simulink model "openloop_response"  (R2022b)
settings: Solver=ode15s  StartTime=0.0  StopTime=20  RelTol=1e-7  AbsTol=1e-7  EnableMultiTasking=on
InitFcn:
  | datacstr
values from neighbouring files (symbols this model uses):
  c_bar = 0.5    [main.m]
  T_bar = 350    [main.m]
libraries: simulink x1
settings Model: Creator=scattolini  LastModifiedBy=marco
settings SolverCC: AutoScaleAbsTol=off  AlgebraicLoopSolver=TrustRegion
settings DataIOCC: SaveFormat=Array  SignalLoggingSaveFormat=ModelDataLogs  ReturnWorkspaceOutputs=off  SignalLoggingName=sigsOut
settings OptimizationCC: BlockReduction=off  BooleanDataType=off  DefaultParameterBehavior=Inlined  BufferReuse=off  ExpressionDepthLimit=2147483647  InitFltsAndDblsToZero=on  LifeSpan=inf
settings DebuggingCC: SaveWithParameterizedLinksMsg=none  UnderspecifiedInitializationDetection=Classic  MergeDetectMultiDrivingBlocksExec=none  SignalResolutionControl=TryResolveAllWithWarning  MultiTaskDSMMsg=warning  MultiTaskCondExecSysMsg=none  FcnCallInpInsideContextMsg=warning  UnconnectedInputMsg=warning  UnconnectedOutputMsg=warning  UnconnectedLineMsg=warning  StateNameClashWarn=warning  SFUnexpectedBacktrackingDiag=warning  SFNoUnconditionalDefaultTransitionDiag=warning  SFExecutionAtInitializationDiag=none  SFMachineParentedDataDiag=warning  ArithmeticOperatorsInVariantConditions=warning
settings HardwareCC: ProdBitPerPointer=32  ProdBitPerSizeT=32  ProdBitPerPtrDiffT=32  ProdLargestAtomicFloat=None  ProdIntDivRoundTo=Undefined  ProdEndianess=Unspecified  ProdWordSize=32  ProdHWDeviceType=32-bit Generic  TargetUnknown=on
settings ModelReferenceCC: EnableRefExpFcnMdlSchedulingChecks=on  PropagateSignalLabelsOutOfModel=off
settings SFSimCC: SimUseLocalCustomCode=off  CustomCodeUndefinedFunction=UseInterfaceOnly
settings RTWCC: RTWUseLocalCustomCode=off  DLArmComputeVersion=19.05
settings CodeAppCC: StateflowObjectComments=on
settings GRTTargetCC: TargetFcnLib=ansi_tfl_tmw.mat  TargetLangStandard=C89/C90 (ANSI)  CombineOutputUpdateFcns=off  GRTInterface=on
settings ConfigComp: CovMetricSettings=dw  CovSaveCumulativeToWorkspaceVar=on  CovSaveSingleToWorkspaceVar=on  CovExternalEMLEnable=off  CovSFcnEnable=off

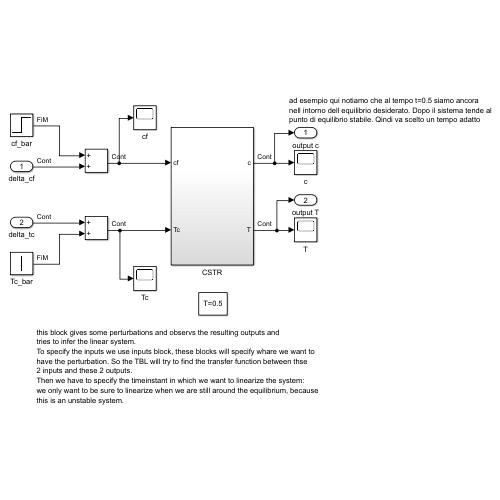
[thumbnail: Simulink's stored preview of the top-level diagram]
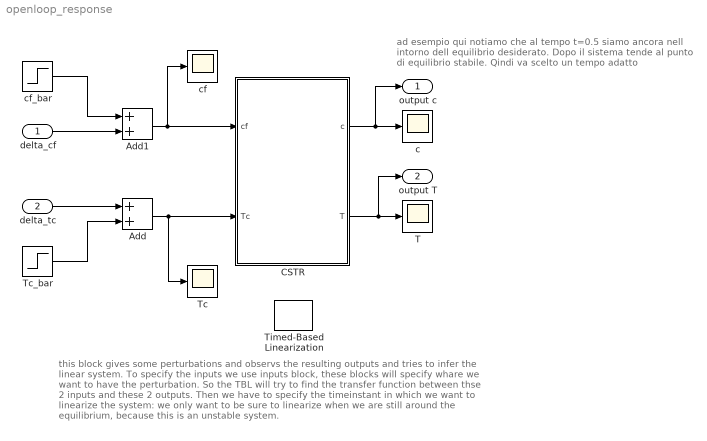
== system openloop_response ==
  note: ad esempio qui notiamo che al tempo t=0.5 siamo ancora
      | nell intorno dell equilibrio desiderato. Dopo il sistema tende al
      | punto di equilibrio stabile. Qindi va scelto un tempo adatto
  note: this block gives some perturbations and observs the resulting outputs and
      | tries to infer the linear system.
      | To specify the inputs we use inputs block, these blocks will specify whare we want to
      | have the perturbation. So the TBL will try to find the transfer function between thse
      | 2 inputs and these 2 outputs.
      | Then we have to specify the timeinstant in which we want to linearize the system:
      | we only want to be sure to linearize when we are still around the equilibrium, because
      | this is an unstable system.
  delta_cf : Inport
  delta_tc : Inport  Port=2
  Add : Sum
  Add1 : Sum
  CSTR : Subsystem
      settings: AttributesFormatString=%<Description>
  T : Scope
  Tc : Scope
  Tc_bar : Step  Time=0  Before=300  After=300  SampleTime=0
  Timed-Based Linearization : simulink/Model-Wide Utilities/Timed-Based Linearization  LinearizationTime=0.5  SampleTime=0
  c : Scope
  cf : Scope
  cf_bar : Step  Time=0  Before=1  SampleTime=0
  output c : Outport
  output T : Outport  Port=2
  wires:
  CSTR/2(T) -> output T/1, T/1
  Add/1 -> Tc/1, CSTR/2(Tc)
  Add1/1 -> cf/1, CSTR/1(cf)
  Tc_bar/1 -> Add/2
  cf_bar/1 -> Add1/1
  CSTR/1(c) -> c/1, output c/1
  delta_cf/1 -> Add1/2
  delta_tc/1 -> Add/1

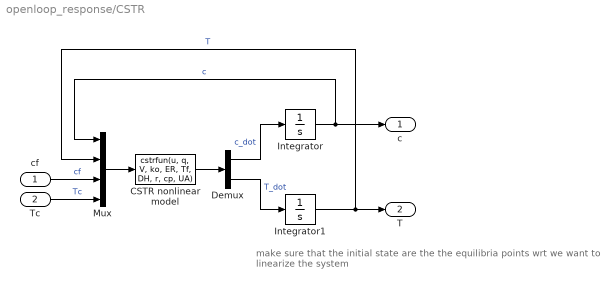
== system openloop_response/CSTR ==
  note: make sure that the initial state are the the equilibria points wrt we want
      | to linearize the system
  cf : Inport
  Tc : Inport  Port=2
  CSTR nonlinear model : MATLABFcn  MATLABFcn=cstrfun(u, q, V, ko, ER, Tf, DH, r, cp, UA)  OutputDimensions=2
  Demux : Demux  Outputs=2
      settings: DisplayOption=none
  Integrator : Integrator  InitialCondition=c_bar
  Integrator1 : Integrator  InitialCondition=T_bar
  Mux : Mux
  c : Outport
  T : Outport  Port=2
  wires:
  Mux/1 -> CSTR nonlinear model/1
  CSTR nonlinear model/1 -> Demux/1
  Demux/1 -> Integrator/1  "c_dot"
  Demux/2 -> Integrator1/1  "T_dot"
  Integrator1/1 -> Mux/2, T/1  "T"
  Integrator/1 -> c/1, Mux/1  "c"
  cf/1 -> Mux/3  "cf"
  Tc/1 -> Mux/4  "Tc"
